simulink model "automotive_fan_control"  (R2025a)
settings: Solver=FixedStepAuto  StartTime=0.0  StopTime=10.0  FixedStep=0.01  RelTol=1e-3
libraries: simulink x2
settings Model: Creator=nikul  LastModifiedBy=nikul
settings ConfigComp: CovEnable=on  RecordCoverage=on  CovMetricSettings=dcmwe  CovModelRefEnable=on

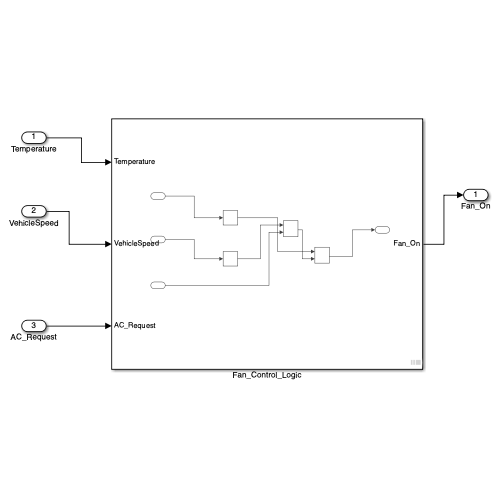
[thumbnail: Simulink's stored preview of the top-level diagram]
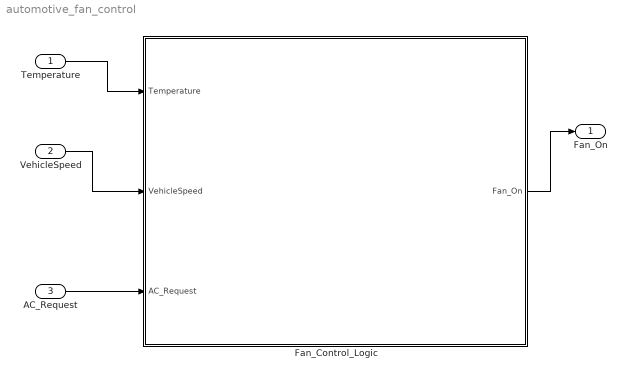
== system automotive_fan_control ==
  Temperature : Inport
  VehicleSpeed : Inport  Port=2
  AC_Request : Inport  Port=3  OutDataTypeStr=boolean
  Fan_Control_Logic : Subsystem
  Fan_On : Outport
  wires:
  Temperature/1 -> Fan_Control_Logic/1(Temperature)
  VehicleSpeed/1 -> Fan_Control_Logic/2(VehicleSpeed)
  AC_Request/1 -> Fan_Control_Logic/3(AC_Request)
  Fan_Control_Logic/1(Fan_On) -> Fan_On/1

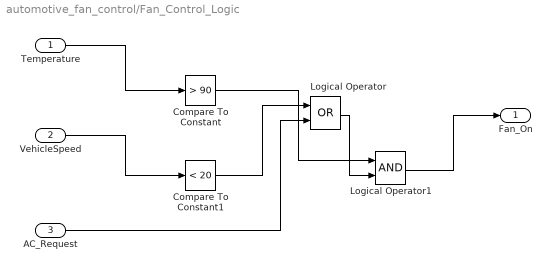
== system automotive_fan_control/Fan_Control_Logic ==
  Temperature : Inport
  VehicleSpeed : Inport  Port=2
  AC_Request : Inport  Port=3
  Compare To Constant : simulink/Logic and Bit Operations/Compare To Constant  relop=>  const=90  OutDataTypeStr=boolean
  Compare To Constant1 : simulink/Logic and Bit Operations/Compare To Constant  relop=<  const=20  OutDataTypeStr=boolean
  Logical Operator : Logic  Operator=OR  AllPortsSameDT=off  OutDataTypeStr=boolean
  Logical Operator1 : Logic  AllPortsSameDT=off  OutDataTypeStr=boolean
  Fan_On : Outport
  wires:
  VehicleSpeed/1 -> Compare To Constant1/1
  Compare To Constant1/1 -> Logical Operator/1
  Logical Operator/1 -> Logical Operator1/2
  Logical Operator1/1 -> Fan_On/1
  Temperature/1 -> Compare To Constant/1
  AC_Request/1 -> Logical Operator/2
  Compare To Constant/1 -> Logical Operator1/1
